simulink model "blokovi2"  (R2014b)
settings: Solver=ode3  StartTime=0.0  StopTime=10.0  RelTol=1e-3
settings Model: Creator=Annie  LastModifiedBy=Annie
settings DataIOCC: SaveFormat=Structure
settings OptimizationCC: UseDivisionForNetSlopeComputation=off  SimCompilerOptimization=off
settings DebuggingCC: SignalResolutionControl=TryResolveAll  FrameProcessingCompatibilityMsg=error
settings RTWCC: RTWCompilerOptimization=off

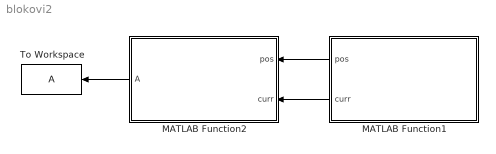
== system blokovi2 ==
  MATLAB Function1 : MATLAB Function  TreatAsAtomicUnit=on
  MATLAB Function2 : MATLAB Function  TreatAsAtomicUnit=on
  To Workspace : ToWorkspace  VariableName=A  SampleTime=-1
  wires:
  MATLAB Function1/1(pos) -> MATLAB Function2/1(pos)
  MATLAB Function1/2(curr) -> MATLAB Function2/2(curr)
  MATLAB Function2/1(A) -> To Workspace/1

== matlab function blokovi2/MATLAB Function2 ==
  data: pos input; curr input; A output
function A  = scenario(pos, curr)
%#codegen
%radijus komunikacije
r = 5;

n=length(pos);
%[m,n] = size(pos);
%inicijalizacija matrice A
A=zeros(n);

for i = 1:n
    for j = 1:n
        %odredivanje udaljenosti izmedju musula - prvo x, y, pa z
        distance = sqrt((pos(1,i)-pos(1,j))^2 + (pos(2,i)-pos(2,j))^2+(pos(3,i)-pos(3,j))^2);
        
        %provjera mogu li komunicirati
        if distance < r
            
            %element ne komunicira sam sa sobom
            if i == j
                A(i,j) = 0;
            else
                A(i,j) = 1;
            end
                        
        else
            A(i,j) = 0;
        end
        
    end
       
end
end

== matlab function blokovi2/MATLAB Function1 ==
  data: pos output; curr output
function [pos, curr] = mussels
%#codegen
%u inpute bi trebalo dodati koordinate, deltu i zetu?

n=5;
pos = zeros (3, n);

X = zeros(1,n);
Y = zeros(1,n);
Z = zeros(1,n);

%mussels su blizu jedna druge

X(1) = 1;
Y(1) = 1;
Z = zeros(1,n);

for i = 2 : n
    
    X(i) = X(i-1)+0.1;
    Y(i) = Y(i-1)+0.1;

end

%mussels su rasprsene

%{
X(1) = 1;
Y(1) = 1;
Z = zeros(1,n);

for i = 2 : n
    
    X(i) = X(i-1)+10;
    Y(i) = Y(i-1)+10;

end
%}

%{
%random postavljanje koordinata
X = randperm(15,n); 
Y = randperm(15,n);
Z = zeros(1,n);
%}

%stvaranje matrice pozicije
    pos(1,:) = X;
    pos(2,:) = Y;
    pos(3,:) = Z;

%mjerenja
curr = randi(3,size(X));

end
